simulink model "gm_HDL_pfc_gold_fi_og_vnl"  (R2024b)
settings: Solver=FixedStepDiscrete  StartTime=0.0  StopTime=.2  RelTol=1e-3
InitFcn:
  | fidelity_pfc_vals;
  | nbits=(2^12)-2;
  | load('C:\Users\Angel\Desktop\hil\pfc3ph\matlab\sim\sschdl\pfc_desktop\stateSpaceParameters.mat');
undefined symbols (not defined in the file or in its folder): a, b, c, DiscIntNeverNeededParam, fsw, Gs, s, stateSpaceParameters_1, t_ss, tsw
libraries: simulink x47, hdlmdlgenlib x24, hdlsllib x10, mcbcontrolslib x5, dspsrcs4 x3, slpidlib x2, hdlssclib x2, spsSVPWMGenerator2LevelLib x1, spsPLL3phLib x1, fillib x1
(part 1 of 5)
settings Model: Creator=angro  LastModifiedBy=Angel
settings OptimizationCC: BlockReduction=off  ConditionallyExecuteInputs=off  DefaultParameterBehavior=Inlined  InheritOutputTypeSmallerThanSingle=on  DefaultUnderspecifiedDataType=single
settings DebuggingCC: SignalRangeChecking=warning  AlgebraicLoopMsg=none  ArtificialAlgebraicLoopMsg=error  InheritedTsInSrcMsg=none  SingleTaskRateTransMsg=error  UnconnectedInputMsg=warning  UnconnectedOutputMsg=warning  UnconnectedLineMsg=warning
settings HardwareCC: ProdBitPerPointer=32  ProdBitPerSizeT=32  ProdBitPerPtrDiffT=32  ProdLargestAtomicFloat=None  ProdIntDivRoundTo=Undefined  ProdEndianess=Unspecified  ProdWordSize=32  ProdHWDeviceType=ASIC/FPGA->ASIC/FPGA  TargetBitPerPointer=64  TargetBitPerSizeT=64  TargetBitPerPtrDiffT=64  TargetLongLongMode=on  TargetIntDivRoundTo=Zero  TargetEndianess=LittleEndian  TargetWordSize=64  TargetHWDeviceType=Custom Processor->MATLAB Host Computer  ProdEqTarget=off

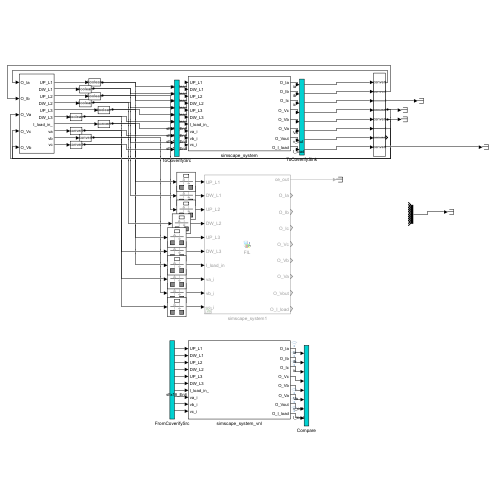
[thumbnail: Simulink's stored preview of the top-level diagram]
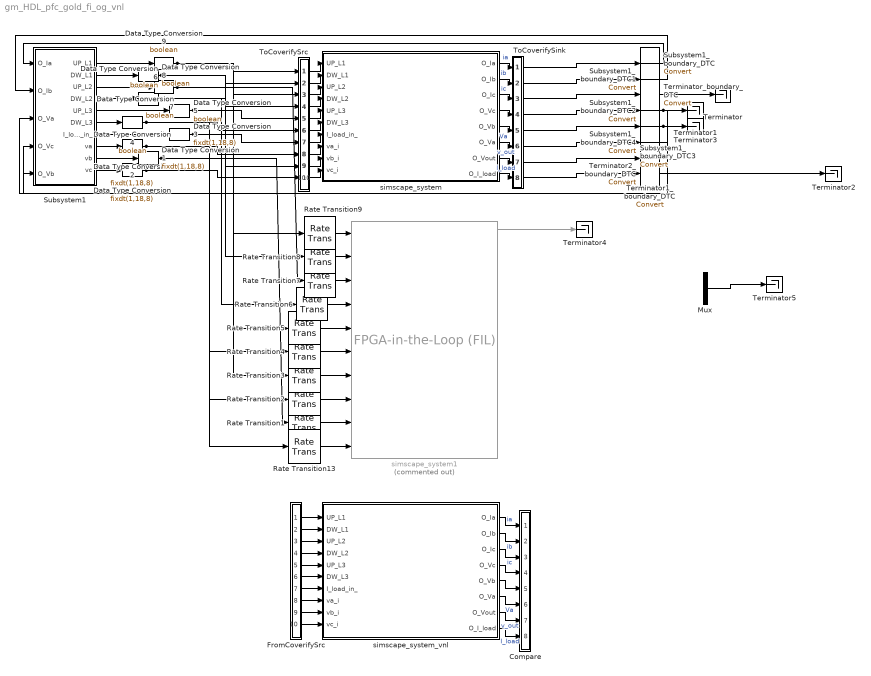
== system gm_HDL_pfc_gold_fi_og_vnl ==
  Compare : Subsystem
      mask Display: disp('')
  Data Type Conversion{,1..3} (4 alike) : DataTypeConversion  OutDataTypeStr=fixdt(1,18,8)  SaturateOnIntegerOverflow=off  RndMeth=Floor
  Data Type Conversion{4..9} (6 alike) : DataTypeConversion  OutDataTypeStr=boolean  SaturateOnIntegerOverflow=off  RndMeth=Floor
  FromCoverifySrc : Subsystem
      mask Display: disp('')
  Mux : Mux  Inputs=9
  Rate Transition{1..9,13} (10 alike) : RateTransition
  Subsystem1 : Subsystem
  Subsystem1_boundary_DTC{,1..4} (5 alike) : DataTypeConversion
  Terminator{,1..5} (6 alike) : Terminator
  Terminator1_boundary_DTC : DataTypeConversion
  Terminator2_boundary_DTC : DataTypeConversion
  Terminator_boundary_DTC : DataTypeConversion
  ToCoverifySink : Subsystem
      mask Display: disp('')
  ToCoverifySrc : Subsystem
      mask Display: disp('')
  simscape_system : Subsystem
  simscape_system1 : fillib/FPGA-in-the-Loop (FIL)  Commented=on  ForceInterfaceUpdate=0.086758
  simscape_system_vnl : Subsystem
  wires:
  Subsystem1/7(I_load_in_) -> Data Type Conversion3/1
  Subsystem1/1(UP_L1) -> Data Type Conversion9/1
  Subsystem1/2(DW_L1) -> Data Type Conversion8/1
  Subsystem1/3(UP_L2) -> Data Type Conversion7/1
  Subsystem1/4(DW_L2) -> Data Type Conversion6/1
  Subsystem1/5(UP_L3) -> Data Type Conversion5/1
  Subsystem1/6(DW_L3) -> Data Type Conversion4/1
  Subsystem1/8(va) -> Data Type Conversion2/1
  Subsystem1/9(vb) -> Data Type Conversion1/1
  Subsystem1/10(vc) -> Data Type Conversion/1
  Data Type Conversion/1 -> Rate Transition13/1, ToCoverifySrc/10(in10)
  Data Type Conversion1/1 -> Rate Transition1/1, ToCoverifySrc/9(in9)
  Data Type Conversion2/1 -> Rate Transition2/1, ToCoverifySrc/8(in8)
  Data Type Conversion3/1 -> Rate Transition3/1, ToCoverifySrc/7(in7)
  Data Type Conversion4/1 -> Rate Transition4/1, ToCoverifySrc/6(in6)
  Data Type Conversion5/1 -> Rate Transition5/1, ToCoverifySrc/5(in5)
  Data Type Conversion6/1 -> Rate Transition6/1, ToCoverifySrc/4(in4)
  Data Type Conversion7/1 -> Rate Transition7/1, ToCoverifySrc/3(in3)
  Data Type Conversion8/1 -> Rate Transition8/1, ToCoverifySrc/2(in2)
  Data Type Conversion9/1 -> Rate Transition9/1, ToCoverifySrc/1(in1)
  Terminator_boundary_DTC/1 -> Terminator/1
  Terminator2_boundary_DTC/1 -> Terminator2/1
  Subsystem1_boundary_DTC/1 -> Subsystem1/1(O_Ia)
  Subsystem1_boundary_DTC1/1 -> Subsystem1/2(O_Ib)
  Subsystem1_boundary_DTC2/1 -> Terminator1/1, Subsystem1/4(O_Vc)
  Subsystem1_boundary_DTC3/1 -> Terminator3/1, Subsystem1/5(O_Vb)
  Subsystem1_boundary_DTC4/1 -> Subsystem1/3(O_Va)
  simscape_system1/1 -> Terminator4/1
  Rate Transition13/1 -> simscape_system1/10
  Rate Transition1/1 -> simscape_system1/9
  Rate Transition2/1 -> simscape_system1/8
  Rate Transition3/1 -> simscape_system1/7
  Rate Transition4/1 -> simscape_system1/6
  Rate Transition5/1 -> simscape_system1/5
  Rate Transition6/1 -> simscape_system1/4
  Rate Transition7/1 -> simscape_system1/3
  Rate Transition8/1 -> simscape_system1/2
  Rate Transition9/1 -> simscape_system1/1
  Mux/1 -> Terminator5/1
  ToCoverifySrc/1(out1) -> simscape_system/1(UP_L1)
  ToCoverifySrc/2(out2) -> simscape_system/2(DW_L1)
  ToCoverifySrc/3(out3) -> simscape_system/3(UP_L2)
  ToCoverifySrc/4(out4) -> simscape_system/4(DW_L2)
  ToCoverifySrc/5(out5) -> simscape_system/5(UP_L3)
  ToCoverifySrc/6(out6) -> simscape_system/6(DW_L3)
  ToCoverifySrc/7(out7) -> simscape_system/7(I_load_in_)
  ToCoverifySrc/8(out8) -> simscape_system/8(va_i)
  ToCoverifySrc/9(out9) -> simscape_system/9(vb_i)
  ToCoverifySrc/10(out10) -> simscape_system/10(vc_i)
  simscape_system/1(O_Ia) -> ToCoverifySink/1(in1)  "ia"
  simscape_system/2(O_Ib) -> ToCoverifySink/2(in2)  "ib"
  simscape_system/3(O_Ic) -> ToCoverifySink/3(in3)  "ic"
  simscape_system/4(O_Vc) -> ToCoverifySink/4(in4)
  simscape_system/5(O_Vb) -> ToCoverifySink/5(in5)
  simscape_system/6(O_Va) -> ToCoverifySink/6(in6)  "Va"
  simscape_system/7(O_Vout) -> ToCoverifySink/7(in7)  "v_out"
  simscape_system/8(O_I_load) -> ToCoverifySink/8(in8)  "I_load"
  ToCoverifySink/1(out1) -> Subsystem1_boundary_DTC/1
  ToCoverifySink/2(out2) -> Subsystem1_boundary_DTC1/1
  ToCoverifySink/3(out3) -> Terminator_boundary_DTC/1
  ToCoverifySink/4(out4) -> Subsystem1_boundary_DTC2/1
  ToCoverifySink/5(out5) -> Subsystem1_boundary_DTC3/1
  ToCoverifySink/6(out6) -> Subsystem1_boundary_DTC4/1
  ToCoverifySink/7(out7) -> Terminator1_boundary_DTC/1
  ToCoverifySink/8(out8) -> Terminator2_boundary_DTC/1
  FromCoverifySrc/1(out1) -> simscape_system_vnl/1(UP_L1)
  FromCoverifySrc/2(out2) -> simscape_system_vnl/2(DW_L1)
  FromCoverifySrc/3(out3) -> simscape_system_vnl/3(UP_L2)
  FromCoverifySrc/4(out4) -> simscape_system_vnl/4(DW_L2)
  FromCoverifySrc/5(out5) -> simscape_system_vnl/5(UP_L3)
  FromCoverifySrc/6(out6) -> simscape_system_vnl/6(DW_L3)
  FromCoverifySrc/7(out7) -> simscape_system_vnl/7(I_load_in_)
  FromCoverifySrc/8(out8) -> simscape_system_vnl/8(va_i)
  FromCoverifySrc/9(out9) -> simscape_system_vnl/9(vb_i)
  FromCoverifySrc/10(out10) -> simscape_system_vnl/10(vc_i)
  simscape_system_vnl/1(O_Ia) -> Compare/1(in1)  "ia"
  simscape_system_vnl/2(O_Ib) -> Compare/2(in2)  "ib"
  simscape_system_vnl/3(O_Ic) -> Compare/3(in3)  "ic"
  simscape_system_vnl/4(O_Vc) -> Compare/4(in4)
  simscape_system_vnl/5(O_Vb) -> Compare/5(in5)
  simscape_system_vnl/6(O_Va) -> Compare/6(in6)  "Va"
  simscape_system_vnl/7(O_Vout) -> Compare/7(in7)  "v_out"
  simscape_system_vnl/8(O_I_load) -> Compare/8(in8)  "I_load"

== system gm_HDL_pfc_gold_fi_og_vnl/Compare ==
  in1 : Inport
  in2 : Inport  Port=2
  in3 : Inport  Port=3
  in4 : Inport  Port=4
  in5 : Inport  Port=5
  in6 : Inport  Port=6
  in7 : Inport  Port=7
  in8 : Inport  Port=8
  Assert_O_I_load : Subsystem
  Assert_O_Ia : Subsystem
  Assert_O_Ib : Subsystem
  Assert_O_Ic : Subsystem
  Assert_O_Va : Subsystem
  Assert_O_Vb : Subsystem
  Assert_O_Vc : Subsystem
  Assert_O_Vout : Subsystem
  CleanupScopes : Subsystem
      settings: OpenFcn=|
      | blkName = gcb; %self block
      | idx = regexp(blkName, '/CleanupScopes$', 'once');
      | blkParent = blkName(1:idx-1);
      | blks=find_system(blkParent, 'LookUnderMasks', 'all','blocktype', 'Scope');
      | for itr = 1:length(blks)
      | 	 hScopeCfg = get_param(blks{itr},'ScopeConfiguration');
      | 	 hScopeCfg.Visible = ~ hScopeCfg.Visible;
      | end
      | drawnow;
      mask Display: fprintf(message('hdlcoder:cosim:vnl_dblclick').getString());
  Enable : Subsystem
      settings: OpenFcn=|
      | blkName = gcb;
      | idx = regexp(blkName, '/Enable$', 'once');
      | blkParent = blkName(1:idx-1);
      | blks=find_system(blkParent, 'LookUnderMasks', 'all','blocktype', 'Assertion');
      | e = get_param(blks{1}, 'Enabled');
      | if strcmp(e, 'on'), f= 'off';, else, f = 'on';, end
      | for ii=1:length(blks), set_param(blks{ii}, 'Enabled', f);, end
      | set_param(gcb, 'MaskDisplay',['fprintf(message(''hdlcoder:cosim:vnl_dblclick_assertions'',','''',upper(e),'''',').getString())']);
      mask Display: fprintf(message('hdlcoder:cosim:vnl_dblclick_assertions','OFF').getString());
  wires:
  in1/1 -> Assert_O_Ia/1(cosim)
  [out1] -> Assert_O_Ia/2(dut)
  in2/1 -> Assert_O_Ib/1(cosim)
  [out2] -> Assert_O_Ib/2(dut)
  in3/1 -> Assert_O_Ic/1(cosim)
  [out3] -> Assert_O_Ic/2(dut)
  in4/1 -> Assert_O_Vc/1(cosim)
  [out4] -> Assert_O_Vc/2(dut)
  in5/1 -> Assert_O_Vb/1(cosim)
  [out5] -> Assert_O_Vb/2(dut)
  in6/1 -> Assert_O_Va/1(cosim)
  [out6] -> Assert_O_Va/2(dut)
  in7/1 -> Assert_O_Vout/1(cosim)
  [out7] -> Assert_O_Vout/2(dut)
  in8/1 -> Assert_O_I_load/1(cosim)
  [out8] -> Assert_O_I_load/2(dut)

== system gm_HDL_pfc_gold_fi_og_vnl/FromCoverifySrc ==
  out1 : Outport
  out2 : Outport  Port=2
  out3 : Outport  Port=3
  out4 : Outport  Port=4
  out5 : Outport  Port=5
  out6 : Outport  Port=6
  out7 : Outport  Port=7
  out8 : Outport  Port=8
  out9 : Outport  Port=9
  out10 : Outport  Port=10
  wires:
  [in1] -> out1/1
  [in2] -> out2/1
  [in3] -> out3/1
  [in4] -> out4/1
  [in5] -> out5/1
  [in6] -> out6/1
  [in7] -> out7/1
  [in8] -> out8/1
  [in9] -> out9/1
  [in10] -> out10/1

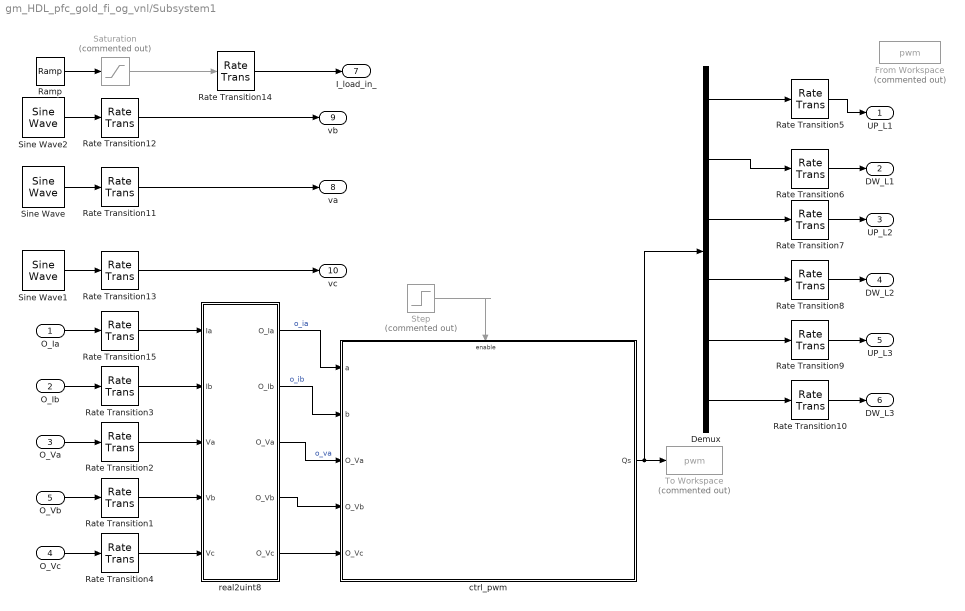
== system gm_HDL_pfc_gold_fi_og_vnl/Subsystem1 ==
  O_Ia : Inport
  O_Ib : Inport  Port=2
  O_Va : Inport  Port=3
  O_Vc : Inport  Port=4
  O_Vb : Inport  Port=5
  Demux : Demux  Outputs=6
  From Workspace : FromWorkspace  Commented=on  VariableName=pwm  SampleTime=t_ss  Interpolate=off  ZeroCross=off  OutputAfterFinalValue=Holding final value
  Ramp : simulink/Sources/Ramp  slope=1/50  start=2/50  InitialOutput=0
  Rate Transition{1..13,15} (14 alike) : RateTransition
  Rate Transition14 : RateTransition  OutPortSampleTime=t_ss
  Saturation : Saturate  Commented=on  UpperLimit=2
  Sine Wave : dspsrcs4/Sine Wave  Amplitude=325  Frequency=50  Phase=0  SampleMode=Discrete  OutComplex=Real  CompMethod=Table lookup  TableSize=Speed  SampleTime=tsw  SamplesPerFrame=1  ResetState=Restart at time zero  OutputFrames=off  dataType=double  wordLen=16  udDataType=sfix(16)  fracBitsMode=Best precision  numFracBits=15  OutDataTypeStr=double  LastOutDataTypeStr=double
  Sine Wave1 : dspsrcs4/Sine Wave  Amplitude=325  Frequency=50  Phase=2*pi/3  SampleMode=Discrete  OutComplex=Real  CompMethod=Table lookup  TableSize=Speed  SampleTime=tsw  SamplesPerFrame=1  ResetState=Restart at time zero  OutputFrames=off  dataType=double  wordLen=16  udDataType=sfix(16)  fracBitsMode=Best precision  numFracBits=15  OutDataTypeStr=double  LastOutDataTypeStr=double
  Sine Wave2 : dspsrcs4/Sine Wave  Amplitude=325  Frequency=50  Phase=-2*pi/3  SampleMode=Discrete  OutComplex=Real  CompMethod=Table lookup  TableSize=Speed  SampleTime=tsw  SamplesPerFrame=1  ResetState=Restart at time zero  OutputFrames=off  dataType=double  wordLen=16  udDataType=sfix(16)  fracBitsMode=Best precision  numFracBits=15  OutDataTypeStr=double  LastOutDataTypeStr=double
  Step : Step  Commented=on  Time=2/50  SampleTime=0
  To Workspace : ToWorkspace  Commented=on  VariableName=pwm  SaveFormat=Timeseries  SampleTime=-1
  ctrl_pwm : Subsystem
  real2uint8 : Subsystem
  UP_L1 : Outport
  DW_L1 : Outport  Port=2
  UP_L2 : Outport  Port=3
  DW_L2 : Outport  Port=4
  UP_L3 : Outport  Port=5
  DW_L3 : Outport  Port=6
  I_load_in_ : Outport  Port=7
  va : Outport  Port=8
  vb : Outport  Port=9
  vc : Outport  Port=10
  wires:
  Ramp/1 -> Saturation/1
  Rate Transition15/1 -> real2uint8/1(Ia)
  Sine Wave2/1 -> Rate Transition12/1
  Saturation/1 -> Rate Transition14/1
  Sine Wave1/1 -> Rate Transition13/1
  Rate Transition8/1 -> DW_L2/1
  Sine Wave/1 -> Rate Transition11/1
  O_Ib/1 -> Rate Transition3/1
  O_Vb/1 -> Rate Transition1/1
  O_Va/1 -> Rate Transition2/1
  O_Ia/1 -> Rate Transition15/1
  O_Vc/1 -> Rate Transition4/1
  Rate Transition2/1 -> real2uint8/3(Va)
  Rate Transition12/1 -> vb/1
  Rate Transition3/1 -> real2uint8/2(Ib)
  Rate Transition11/1 -> va/1
  Rate Transition1/1 -> real2uint8/4(Vb)
  Rate Transition13/1 -> vc/1
  Rate Transition4/1 -> real2uint8/5(Vc)
  Rate Transition10/1 -> DW_L3/1
  Rate Transition14/1 -> I_load_in_/1
  Step/1 -> ctrl_pwm/Enable
  real2uint8/4(O_Vb) -> ctrl_pwm/4(O_Vb)
  real2uint8/1(O_Ia) -> ctrl_pwm/1(a)  "o_ia"
  real2uint8/2(O_Ib) -> ctrl_pwm/2(b)  "o_ib"
  real2uint8/3(O_Va) -> ctrl_pwm/3(O_Va)  "o_va"
  real2uint8/5(O_Vc) -> ctrl_pwm/5(O_Vc)
  ctrl_pwm/1(Qs) -> Demux/1, To Workspace/1
  Demux/5 -> Rate Transition9/1
  Demux/1 -> Rate Transition5/1
  Demux/6 -> Rate Transition10/1
  Demux/2 -> Rate Transition6/1
  Demux/3 -> Rate Transition7/1
  Demux/4 -> Rate Transition8/1
  Rate Transition5/1 -> UP_L1/1
  Rate Transition6/1 -> DW_L1/1
  Rate Transition7/1 -> UP_L2/1
  Rate Transition9/1 -> UP_L3/1

== system gm_HDL_pfc_gold_fi_og_vnl/ToCoverifySink ==
  in1 : Inport
  in2 : Inport  Port=2
  in3 : Inport  Port=3
  in4 : Inport  Port=4
  in5 : Inport  Port=5
  in6 : Inport  Port=6
  in7 : Inport  Port=7
  in8 : Inport  Port=8
  out1 : Outport
  out2 : Outport  Port=2
  out3 : Outport  Port=3
  out4 : Outport  Port=4
  out5 : Outport  Port=5
  out6 : Outport  Port=6
  out7 : Outport  Port=7
  out8 : Outport  Port=8
  tag scope: out1=global, out2=global, out3=global, out4=global, out5=global, out6=global, out7=global, out8=global
  wires:
  in1/1 -> out1/1, [out1]
  in2/1 -> out2/1, [out2]
  in3/1 -> out3/1, [out3]
  in4/1 -> out4/1, [out4]
  in5/1 -> out5/1, [out5]
  in6/1 -> out6/1, [out6]
  in7/1 -> out7/1, [out7]
  in8/1 -> out8/1, [out8]

== system gm_HDL_pfc_gold_fi_og_vnl/ToCoverifySrc ==
  in1 : Inport
  in2 : Inport  Port=2
  in3 : Inport  Port=3
  in4 : Inport  Port=4
  in5 : Inport  Port=5
  in6 : Inport  Port=6
  in7 : Inport  Port=7
  in8 : Inport  Port=8
  in9 : Inport  Port=9
  in10 : Inport  Port=10
  out1 : Outport
  out2 : Outport  Port=2
  out3 : Outport  Port=3
  out4 : Outport  Port=4
  out5 : Outport  Port=5
  out6 : Outport  Port=6
  out7 : Outport  Port=7
  out8 : Outport  Port=8
  out9 : Outport  Port=9
  out10 : Outport  Port=10
  tag scope: in10=global, in1=global, in2=global, in3=global, in4=global, in5=global, in6=global, in7=global, in8=global, in9=global
  wires:
  in1/1 -> out1/1, [in1]
  in2/1 -> out2/1, [in2]
  in3/1 -> out3/1, [in3]
  in4/1 -> out4/1, [in4]
  in5/1 -> out5/1, [in5]
  in6/1 -> out6/1, [in6]
  in7/1 -> out7/1, [in7]
  in8/1 -> out8/1, [in8]
  in9/1 -> out9/1, [in9]
  in10/1 -> out10/1, [in10]

== system gm_HDL_pfc_gold_fi_og_vnl/simscape_system ==
  UP_L1 : Inport  OutDataTypeStr=boolean  PortDimensions=1  SampleTime=5.12820512820513e-07
  DW_L1 : Inport  Port=2  OutDataTypeStr=boolean  PortDimensions=1  SampleTime=5.12820512820513e-07
  UP_L2 : Inport  Port=3  OutDataTypeStr=boolean  PortDimensions=1  SampleTime=5.12820512820513e-07
  DW_L2 : Inport  Port=4  OutDataTypeStr=boolean  PortDimensions=1  SampleTime=5.12820512820513e-07
  UP_L3 : Inport  Port=5  OutDataTypeStr=boolean  PortDimensions=1  SampleTime=5.12820512820513e-07
  DW_L3 : Inport  Port=6  OutDataTypeStr=boolean  PortDimensions=1  SampleTime=5.12820512820513e-07
  I_load_in_ : Inport  Port=7  OutDataTypeStr=fixdt(1, 18, 8)  PortDimensions=1  SampleTime=5.12820512820513e-07
  va_i : Inport  Port=8  OutDataTypeStr=fixdt(1, 18, 8)  PortDimensions=1  SampleTime=5.12820512820513e-07  LockScale=on
  vb_i : Inport  Port=9  OutDataTypeStr=fixdt(1, 18, 8)  PortDimensions=1  SampleTime=5.12820512820513e-07  LockScale=on
  vc_i : Inport  Port=10  OutDataTypeStr=fixdt(1, 18, 8)  PortDimensions=1  SampleTime=5.12820512820513e-07  LockScale=on
  simscape_system : Subsystem
  t{,1..7} (8 alike) : RateTransition  InitialCondition=double(0)  OutPortSampleTimeOpt=Multiple of input port sample time  OutPortSampleTimeMultiple=37
  O_Ia : Outport  SampleTime=5.12820512820513e-07
  O_Ib : Outport  Port=2  SampleTime=5.12820512820513e-07
  O_Ic : Outport  Port=3  SampleTime=5.12820512820513e-07
  O_Vc : Outport  Port=4  SampleTime=5.12820512820513e-07
  O_Vb : Outport  Port=5  SampleTime=5.12820512820513e-07
  O_Va : Outport  Port=6  SampleTime=5.12820512820513e-07
  O_Vout : Outport  Port=7  SampleTime=5.12820512820513e-07
  O_I_load : Outport  Port=8  SampleTime=5.12820512820513e-07
  wires:
  t6/1 -> O_I_load/1
  t5/1 -> O_Vout/1
  t4/1 -> O_Va/1
  t3/1 -> O_Vb/1
  t2/1 -> O_Vc/1
  t1/1 -> O_Ic/1
  t/1 -> O_Ib/1
  t7/1 -> O_Ia/1
  simscape_system/8(O_I_load) -> t6/1
  simscape_system/7(O_Vout) -> t5/1
  simscape_system/6(O_Va) -> t4/1
  simscape_system/5(O_Vb) -> t3/1
  simscape_system/4(O_Vc) -> t2/1
  simscape_system/3(O_Ic) -> t1/1
  simscape_system/2(O_Ib) -> t/1
  simscape_system/1(O_Ia) -> t7/1
  vc_i/1 -> simscape_system/10(vc_i)
  vb_i/1 -> simscape_system/9(vb_i)
  I_load_in_/1 -> simscape_system/7(I_load_in_)
  va_i/1 -> simscape_system/8(va_i)
  UP_L1/1 -> simscape_system/1(UP_L1)
  DW_L1/1 -> simscape_system/2(DW_L1)
  UP_L2/1 -> simscape_system/3(UP_L2)
  DW_L2/1 -> simscape_system/4(DW_L2)
  UP_L3/1 -> simscape_system/5(UP_L3)
  DW_L3/1 -> simscape_system/6(DW_L3)

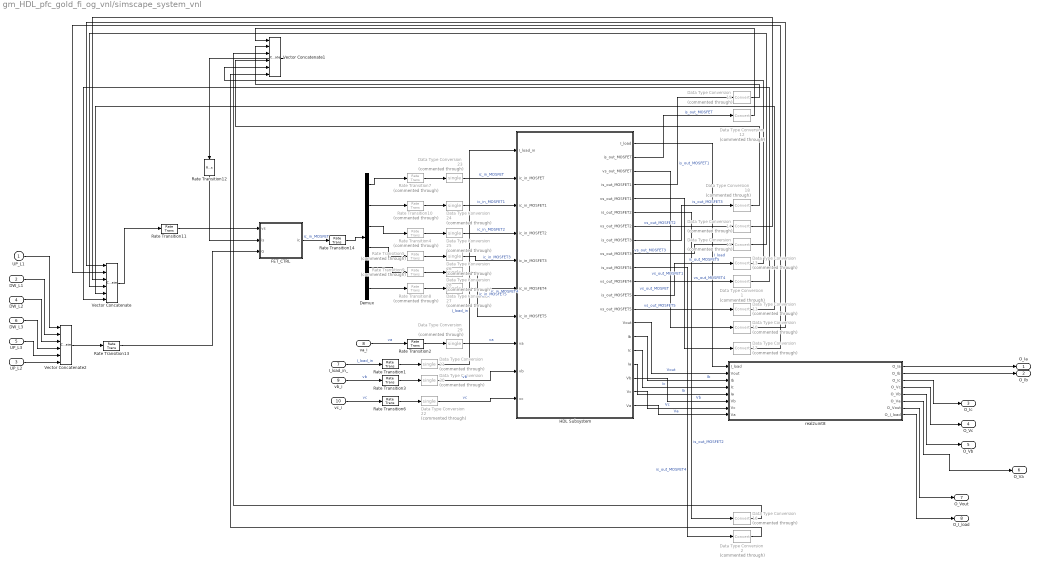
== system gm_HDL_pfc_gold_fi_og_vnl/simscape_system_vnl ==
  UP_L1 : Inport
  DW_L1 : Inport  Port=2
  UP_L2 : Inport  Port=3
  DW_L2 : Inport  Port=4
  UP_L3 : Inport  Port=5
  DW_L3 : Inport  Port=6
  I_load_in_ : Inport  Port=7  OutDataTypeStr=fixdt(1,18,8)
  va_i : Inport  Port=8  LockScale=on
  vb_i : Inport  Port=9  LockScale=on
  vc_i : Inport  Port=10  LockScale=on
  Data Type Conversion{1..2,10..19} (12 alike) : DataTypeConversion  Commented=through  RndMeth=Nearest  SaturateOnIntegerOverflow=off  LockScale=on
  Data Type Conversion{21..30} (10 alike) : DataTypeConversion  Commented=through  OutDataTypeStr=single  RndMeth=Nearest  SaturateOnIntegerOverflow=off
  Demux : Demux  Outputs=6
  FET_CTRL : Subsystem
  HDL Subsystem : Subsystem
  Rate Transition{1..3,6,11..13} (7 alike) : RateTransition  OutPortSampleTime=t_ss
  Rate Transition{4..5,7..10} (6 alike) : RateTransition  Commented=through  OutPortSampleTime=t_ss
  Rate Transition14 : RateTransition  Integrity=off  OutPortSampleTime=t_ss
  Vector Concatenate : Concatenate  NumInputs=6
  Vector Concatenate1 : Concatenate  NumInputs=6
  Vector Concatenate2 : Concatenate  NumInputs=6
  real2uint8 : Subsystem
  O_Ia : Outport
  O_Ib : Outport  Port=2
  O_Ic : Outport  Port=3
  O_Vc : Outport  Port=4
  O_Vb : Outport  Port=5
  O_Va : Outport  Port=6
  O_Vout : Outport  Port=7
  O_I_load : Outport  Port=8
  wires:
  real2uint8/6(O_Va) -> O_Va/1
  real2uint8/2(O_Ib) -> O_Ib/1
  real2uint8/1(O_Ia) -> O_Ia/1
  Rate Transition12/1 -> FET_CTRL/2(is)
  Rate Transition11/1 -> FET_CTRL/1(vs)
  Rate Transition14/1 -> Demux/1
  Vector Concatenate1/1 -> Rate Transition12/1
  Vector Concatenate/1 -> Rate Transition11/1
  Rate Transition13/1 -> FET_CTRL/3(G)
  real2uint8/7(O_Vout) -> O_Vout/1
  Data Type Conversion2/1 -> Vector Concatenate1/6
  Data Type Conversion16/1 -> Vector Concatenate1/3
  real2uint8/8(O_I_load) -> O_I_load/1
  real2uint8/5(O_Vb) -> O_Vb/1
  real2uint8/4(O_Vc) -> O_Vc/1
  real2uint8/3(O_Ic) -> O_Ic/1
  Data Type Conversion17/1 -> Vector Concatenate/2
  Data Type Conversion10/1 -> Vector Concatenate/1
  Data Type Conversion11/1 -> Vector Concatenate/5
  Data Type Conversion1/1 -> Vector Concatenate/6
  Data Type Conversion13/1 -> Vector Concatenate1/5
  Data Type Conversion15/1 -> Vector Concatenate/4
  Data Type Conversion14/1 -> Vector Concatenate/3
  Data Type Conversion12/1 -> Vector Concatenate1/1
  HDL Subsystem/11(vs_out_MOSFET4) -> Data Type Conversion1/1  "vs_out_MOSFET4"
  HDL Subsystem/12(is_out_MOSFET5) -> Data Type Conversion13/1  "is_out_MOSFET5"
  HDL Subsystem/9(vs_out_MOSFET3) -> Data Type Conversion15/1  "vs_out_MOSFET3"
  HDL Subsystem/10(is_out_MOSFET4) -> Data Type Conversion2/1  "is_out_MOSFET4"
  HDL Subsystem/7(vs_out_MOSFET2) -> Data Type Conversion14/1  "vs_out_MOSFET2"
  HDL Subsystem/8(is_out_MOSFET3) -> Data Type Conversion18/1  "is_out_MOSFET3"
  HDL Subsystem/5(vs_out_MOSFET1) -> Data Type Conversion17/1  "vs_out_MOSFET1"
  HDL Subsystem/6(is_out_MOSFET2) -> Data Type Conversion16/1  "is_out_MOSFET2"
  Data Type Conversion22/1 -> HDL Subsystem/10(vc)  "vc"
  Data Type Conversion30/1 -> HDL Subsystem/9(vb)  "vb"
  HDL Subsystem/3(vs_out_MOSFET) -> Data Type Conversion10/1  "vs_out_MOSFET"
  HDL Subsystem/4(is_out_MOSFET1) -> Data Type Conversion19/1  "is_out_MOSFET1"
  Data Type Conversion29/1 -> HDL Subsystem/8(va)  "va"
  Data Type Conversion27/1 -> HDL Subsystem/6(ic_in_MOSFET4)  "ic_in_MOSFET4"
  Data Type Conversion28/1 -> HDL Subsystem/7(ic_in_MOSFET5)  "ic_in_MOSFET5"
  Data Type Conversion26/1 -> HDL Subsystem/5(ic_in_MOSFET3)  "ic_in_MOSFET3"
  Data Type Conversion25/1 -> HDL Subsystem/4(ic_in_MOSFET2)  "ic_in_MOSFET2"
  Data Type Conversion23/1 -> HDL Subsystem/2(ic_in_MOSFET)  "ic_in_MOSFET"
  Rate Transition6/1 -> Data Type Conversion22/1
  Data Type Conversion19/1 -> Vector Concatenate1/2
  Rate Transition3/1 -> Data Type Conversion30/1
  Rate Transition1/1 -> Data Type Conversion21/1
  Data Type Conversion24/1 -> HDL Subsystem/3(ic_in_MOSFET1)  "ic_in_MOSFET1"
  Rate Transition2/1 -> Data Type Conversion29/1
  Data Type Conversion18/1 -> Vector Concatenate1/4
  Rate Transition8/1 -> Data Type Conversion27/1
  Rate Transition9/1 -> Data Type Conversion28/1
  Data Type Conversion21/1 -> HDL Subsystem/1(I_load_in)  "I_load_in"
  Rate Transition5/1 -> Data Type Conversion26/1
  Rate Transition4/1 -> Data Type Conversion25/1
  Rate Transition10/1 -> Data Type Conversion24/1
  vc_i/1 -> Rate Transition6/1  "vc"
  Demux/5 -> Rate Transition9/1
  Demux/6 -> Rate Transition8/1
  vb_i/1 -> Rate Transition3/1  "vb"
  Demux/3 -> Rate Transition4/1
  Demux/4 -> Rate Transition5/1
  va_i/1 -> Rate Transition2/1  "va"
  Rate Transition7/1 -> Data Type Conversion23/1
  Demux/1 -> Rate Transition7/1
  Demux/2 -> Rate Transition10/1
  I_load_in_/1 -> Rate Transition1/1  "I_load_in"
  FET_CTRL/1(ic) -> Rate Transition14/1  "ic_in_MOSFET"
  Vector Concatenate2/1 -> Rate Transition13/1
  HDL Subsystem/1(I_load) -> real2uint8/1(I_load)  "I_load"
  HDL Subsystem/2(is_out_MOSFET) -> Data Type Conversion12/1  "is_out_MOSFET"
  UP_L2/1 -> Vector Concatenate2/6
  HDL Subsystem/17(Ia) -> real2uint8/5(Ia)  "Ia"
  HDL Subsystem/18(Vb) -> real2uint8/6(Vb)  "Vb"
  UP_L3/1 -> Vector Concatenate2/5
  DW_L3/1 -> Vector Concatenate2/4
  DW_L2/1 -> Vector Concatenate2/3
  HDL Subsystem/19(Vc) -> real2uint8/7(Vc)  "Vc"
  HDL Subsystem/20(Va) -> real2uint8/8(Va)  "Va"
  DW_L1/1 -> Vector Concatenate2/2
  HDL Subsystem/15(Ib) -> real2uint8/3(Ib)  "Ib"
  HDL Subsystem/16(Ic) -> real2uint8/4(Ic)  "Ic"
  UP_L1/1 -> Vector Concatenate2/1
  HDL Subsystem/13(vs_out_MOSFET5) -> Data Type Conversion11/1  "vs_out_MOSFET5"
  HDL Subsystem/14(Vout) -> real2uint8/2(Vout)  "Vout"

== system gm_HDL_pfc_gold_fi_og_vnl/Compare/Assert_O_I_load ==
  cosim : Inport
  dut : Inport  Port=2
  AssertEq : Assertion  StopWhenAssertionFail=off
  Compare To Zero : simulink/Logic and Bit Operations/Compare To Zero  relop===  OutDataTypeStr=boolean
  Relational Operator : RelationalOperator  Operator===  OutDataTypeStr=boolean  InputSameDT=off
  compare: O_I_load : Scope  NumInputPorts=3
  wires:
  Compare To Zero/1 -> compare: O_I_load/3  "err"
  Relational Operator/1 -> Compare To Zero/1, AssertEq/1
  cosim/1 -> compare: O_I_load/1, Relational Operator/1  "cosim"
  dut/1 -> compare: O_I_load/2, Relational Operator/2  "dut ref"

== system gm_HDL_pfc_gold_fi_og_vnl/Compare/Assert_O_Ia ==
  cosim : Inport
  dut : Inport  Port=2
  AssertEq : Assertion  StopWhenAssertionFail=off
  Compare To Zero : simulink/Logic and Bit Operations/Compare To Zero  relop===  OutDataTypeStr=boolean
  Relational Operator : RelationalOperator  Operator===  OutDataTypeStr=boolean  InputSameDT=off
  compare: O_Ia : Scope  NumInputPorts=3
  wires:
  Compare To Zero/1 -> compare: O_Ia/3  "err"
  Relational Operator/1 -> Compare To Zero/1, AssertEq/1
  cosim/1 -> compare: O_Ia/1, Relational Operator/1  "cosim"
  dut/1 -> compare: O_Ia/2, Relational Operator/2  "dut ref"

== system gm_HDL_pfc_gold_fi_og_vnl/Compare/Assert_O_Ib ==
  cosim : Inport
  dut : Inport  Port=2
  AssertEq : Assertion  StopWhenAssertionFail=off
  Compare To Zero : simulink/Logic and Bit Operations/Compare To Zero  relop===  OutDataTypeStr=boolean
  Relational Operator : RelationalOperator  Operator===  OutDataTypeStr=boolean  InputSameDT=off
  compare: O_Ib : Scope  NumInputPorts=3
  wires:
  Compare To Zero/1 -> compare: O_Ib/3  "err"
  Relational Operator/1 -> Compare To Zero/1, AssertEq/1
  cosim/1 -> compare: O_Ib/1, Relational Operator/1  "cosim"
  dut/1 -> compare: O_Ib/2, Relational Operator/2  "dut ref"

== system gm_HDL_pfc_gold_fi_og_vnl/Compare/Assert_O_Ic ==
  cosim : Inport
  dut : Inport  Port=2
  AssertEq : Assertion  StopWhenAssertionFail=off
  Compare To Zero : simulink/Logic and Bit Operations/Compare To Zero  relop===  OutDataTypeStr=boolean
  Relational Operator : RelationalOperator  Operator===  OutDataTypeStr=boolean  InputSameDT=off
  compare: O_Ic : Scope  NumInputPorts=3
  wires:
  Compare To Zero/1 -> compare: O_Ic/3  "err"
  Relational Operator/1 -> Compare To Zero/1, AssertEq/1
  cosim/1 -> compare: O_Ic/1, Relational Operator/1  "cosim"
  dut/1 -> compare: O_Ic/2, Relational Operator/2  "dut ref"

== system gm_HDL_pfc_gold_fi_og_vnl/Compare/Assert_O_Va ==
  cosim : Inport
  dut : Inport  Port=2
  AssertEq : Assertion  StopWhenAssertionFail=off
  Compare To Zero : simulink/Logic and Bit Operations/Compare To Zero  relop===  OutDataTypeStr=boolean
  Relational Operator : RelationalOperator  Operator===  OutDataTypeStr=boolean  InputSameDT=off
  compare: O_Va : Scope  NumInputPorts=3
  wires:
  Compare To Zero/1 -> compare: O_Va/3  "err"
  Relational Operator/1 -> Compare To Zero/1, AssertEq/1
  cosim/1 -> compare: O_Va/1, Relational Operator/1  "cosim"
  dut/1 -> compare: O_Va/2, Relational Operator/2  "dut ref"

== system gm_HDL_pfc_gold_fi_og_vnl/Compare/Assert_O_Vb ==
  cosim : Inport
  dut : Inport  Port=2
  AssertEq : Assertion  StopWhenAssertionFail=off
  Compare To Zero : simulink/Logic and Bit Operations/Compare To Zero  relop===  OutDataTypeStr=boolean
  Relational Operator : RelationalOperator  Operator===  OutDataTypeStr=boolean  InputSameDT=off
  compare: O_Vb : Scope  NumInputPorts=3
  wires:
  Compare To Zero/1 -> compare: O_Vb/3  "err"
  Relational Operator/1 -> Compare To Zero/1, AssertEq/1
  cosim/1 -> compare: O_Vb/1, Relational Operator/1  "cosim"
  dut/1 -> compare: O_Vb/2, Relational Operator/2  "dut ref"

== system gm_HDL_pfc_gold_fi_og_vnl/Compare/Assert_O_Vc ==
  cosim : Inport
  dut : Inport  Port=2
  AssertEq : Assertion  StopWhenAssertionFail=off
  Compare To Zero : simulink/Logic and Bit Operations/Compare To Zero  relop===  OutDataTypeStr=boolean
  Relational Operator : RelationalOperator  Operator===  OutDataTypeStr=boolean  InputSameDT=off
  compare: O_Vc : Scope  NumInputPorts=3
  wires:
  Compare To Zero/1 -> compare: O_Vc/3  "err"
  Relational Operator/1 -> Compare To Zero/1, AssertEq/1
  cosim/1 -> compare: O_Vc/1, Relational Operator/1  "cosim"
  dut/1 -> compare: O_Vc/2, Relational Operator/2  "dut ref"

== system gm_HDL_pfc_gold_fi_og_vnl/Compare/Assert_O_Vout ==
  cosim : Inport
  dut : Inport  Port=2
  AssertEq : Assertion  StopWhenAssertionFail=off
  Compare To Zero : simulink/Logic and Bit Operations/Compare To Zero  relop===  OutDataTypeStr=boolean
  Relational Operator : RelationalOperator  Operator===  OutDataTypeStr=boolean  InputSameDT=off
  compare: O_Vout : Scope  NumInputPorts=3
  wires:
  Compare To Zero/1 -> compare: O_Vout/3  "err"
  Relational Operator/1 -> Compare To Zero/1, AssertEq/1
  cosim/1 -> compare: O_Vout/1, Relational Operator/1  "cosim"
  dut/1 -> compare: O_Vout/2, Relational Operator/2  "dut ref"

== system gm_HDL_pfc_gold_fi_og_vnl/Compare/CleanupScopes ==

== system gm_HDL_pfc_gold_fi_og_vnl/Compare/Enable ==

== system gm_HDL_pfc_gold_fi_og_vnl/Subsystem1/ctrl_pwm ==
  a : Inport
  b : Inport  Port=2
  O_Va : Inport  Port=3
  O_Vb : Inport  Port=4
  O_Vc : Inport  Port=5
  Enable : EnablePort
  PI_CTRL : Subsystem
  SVPWM : Subsystem
  transforms : Subsystem
  Qs : Outport
  wires:
  transforms/1(id) -> PI_CTRL/1(id)
  transforms/3(angle) -> SVPWM/2(angle)
  PI_CTRL/1(Vd_inductor) -> SVPWM/1(Vd_inductor)
  a/1 -> transforms/1(a)
  O_Vc/1 -> transforms/5(In5)
  transforms/2(iq) -> PI_CTRL/2(iq)
  SVPWM/1(P) -> Qs/1  "Qs"
  PI_CTRL/2(Vq_inductor) -> SVPWM/3(Vq_inductor)
  b/1 -> transforms/2(b)
  O_Va/1 -> transforms/3(In3)
  O_Vb/1 -> transforms/4(In4)

== system gm_HDL_pfc_gold_fi_og_vnl/Subsystem1/real2uint8 ==
  Ia : Inport
  Ib : Inport  Port=2
  Va : Inport  Port=3
  Vb : Inport  Port=4
  Vc : Inport  Port=5
  Add2 : Sum  Inputs=-+  OutDataTypeStr=Inherit: Same as first input
  Add3 : Sum  Inputs=+-
  Constant : Constant  Value=40  SampleTime=-1
  Constant1 : Constant  Value=420  SampleTime=-1
  Demux : Demux  Outputs=3
  Demux1 : Demux  Outputs=2
  Gain2 : Gain  Gain=80/nbits  OutDataTypeStr=Inherit: Same as input
  Gain5 : Gain  Gain=840/nbits  OutDataTypeStr=Inherit: Same as input
  Mux : Mux  Inputs=3
  Mux1 : Mux  Inputs=2
  O_Ia : Outport
  O_Ib : Outport  Port=2
  O_Va : Outport  Port=3
  O_Vb : Outport  Port=4
  O_Vc : Outport  Port=5
  wires:
  Va/1 -> Mux/3
  Vb/1 -> Mux/1
  Ia/1 -> Mux1/2  "rIA"
  Vc/1 -> Mux/2
  Ib/1 -> Mux1/1
  Demux/1 -> O_Vb/1
  Constant1/1 -> Add3/2
  Constant/1 -> Add2/1
  Demux/2 -> O_Vc/1
  Demux/3 -> O_Va/1
  Demux1/1 -> O_Ib/1
  Demux1/2 -> O_Ia/1
  Mux1/1 -> Gain2/1
  Mux/1 -> Gain5/1
  Gain5/1 -> Add3/1
  Gain2/1 -> Add2/2
  Add2/1 -> Demux1/1
  Add3/1 -> Demux/1

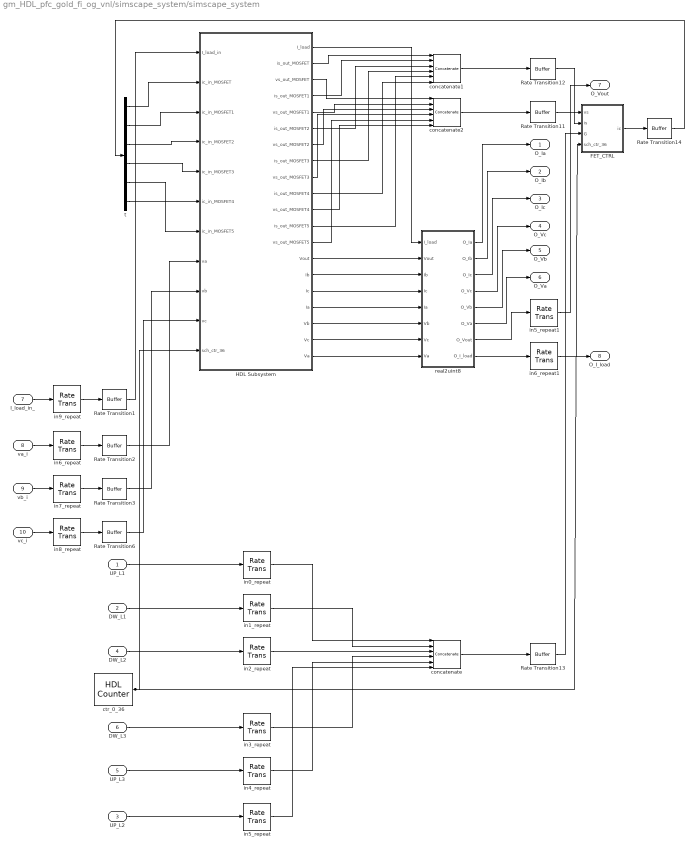
== system gm_HDL_pfc_gold_fi_og_vnl/simscape_system/simscape_system ==
  UP_L1 : Inport  OutDataTypeStr=boolean  SampleTime=5.12820512820513e-07
  DW_L1 : Inport  Port=2  OutDataTypeStr=boolean  SampleTime=5.12820512820513e-07
  UP_L2 : Inport  Port=3  OutDataTypeStr=boolean  SampleTime=5.12820512820513e-07
  DW_L2 : Inport  Port=4  OutDataTypeStr=boolean  SampleTime=5.12820512820513e-07
  UP_L3 : Inport  Port=5  OutDataTypeStr=boolean  SampleTime=5.12820512820513e-07
  DW_L3 : Inport  Port=6  OutDataTypeStr=boolean  SampleTime=5.12820512820513e-07
  I_load_in_ : Inport  Port=7  OutDataTypeStr=fixdt(1, 18, 8)  SampleTime=5.12820512820513e-07
  va_i : Inport  Port=8  OutDataTypeStr=fixdt(1, 18, 8)  SampleTime=5.12820512820513e-07
  vb_i : Inport  Port=9  OutDataTypeStr=fixdt(1, 18, 8)  SampleTime=5.12820512820513e-07
  vc_i : Inport  Port=10  OutDataTypeStr=fixdt(1, 18, 8)  SampleTime=5.12820512820513e-07
  FET_CTRL : Subsystem
  HDL Subsystem : Subsystem
  Rate Transition{1..3,6,11..14} (8 alike) : hdlmdlgenlib/Buffer
  concatenate : Concatenate  NumInputs=6
  concatenate1 : Concatenate  NumInputs=6
  concatenate2 : Concatenate  NumInputs=6
  ctr_0_36 : hdlsllib/Sources/HDL Counter  CountType=Count limited  CountInit=double(0)  CountStep=double(1)  CountMax=double(36)  CountFromType=Initial value  CountFrom=double(0)  CountResetPort=off  CountLoadPort=off  CountEnbPort=off  CountDirPort=off  CountHitOutputPort=off  CountDataType=Unsigned  CountWordLen=6  CountFracLen=0  CountSampTime=1.38600138600139e-08
  in0_repeat : RateTransition  Integrity=off  Deterministic=off  OutPortSampleTimeOpt=Multiple of input port sample time  OutPortSampleTimeMultiple=1/37
  in1_repeat : RateTransition  Integrity=off  Deterministic=off  OutPortSampleTimeOpt=Multiple of input port sample time  OutPortSampleTimeMultiple=1/37
  in2_repeat : RateTransition  Integrity=off  Deterministic=off  OutPortSampleTimeOpt=Multiple of input port sample time  OutPortSampleTimeMultiple=1/37
  in3_repeat : RateTransition  Integrity=off  Deterministic=off  OutPortSampleTimeOpt=Multiple of input port sample time  OutPortSampleTimeMultiple=1/37
  in4_repeat : RateTransition  Integrity=off  Deterministic=off  OutPortSampleTimeOpt=Multiple of input port sample time  OutPortSampleTimeMultiple=1/37
  in5_repeat : RateTransition  Integrity=off  Deterministic=off  OutPortSampleTimeOpt=Multiple of input port sample time  OutPortSampleTimeMultiple=1/37
  in5_repeat1 : RateTransition  Integrity=off  Deterministic=off  OutPortSampleTimeOpt=Multiple of input port sample time  OutPortSampleTimeMultiple=1/37
  in6_repeat : RateTransition  Integrity=off  Deterministic=off  OutPortSampleTimeOpt=Multiple of input port sample time  OutPortSampleTimeMultiple=1/37
  in6_repeat1 : RateTransition  Integrity=off  Deterministic=off  OutPortSampleTimeOpt=Multiple of input port sample time  OutPortSampleTimeMultiple=1/37
  in7_repeat : RateTransition  Integrity=off  Deterministic=off  OutPortSampleTimeOpt=Multiple of input port sample time  OutPortSampleTimeMultiple=1/37
  in8_repeat : RateTransition  Integrity=off  Deterministic=off  OutPortSampleTimeOpt=Multiple of input port sample time  OutPortSampleTimeMultiple=1/37
  in9_repeat : RateTransition  Integrity=off  Deterministic=off  OutPortSampleTimeOpt=Multiple of input port sample time  OutPortSampleTimeMultiple=1/37
  real2uint8 : Subsystem
  t : Demux  Outputs=6
  O_Ia : Outport  OutDataTypeStr=fixdt(0, 12, -1)  SampleTime=1.38600138600139e-08
  O_Ib : Outport  Port=2  OutDataTypeStr=fixdt(0, 12, -1)  SampleTime=1.38600138600139e-08
  O_Ic : Outport  Port=3  OutDataTypeStr=fixdt(0, 12, -1)  SampleTime=1.38600138600139e-08
  O_Vc : Outport  Port=4  OutDataTypeStr=fixdt(0, 12, -1)  SampleTime=1.38600138600139e-08
  O_Vb : Outport  Port=5  OutDataTypeStr=fixdt(0, 12, -1)  SampleTime=1.38600138600139e-08
  O_Va : Outport  Port=6  OutDataTypeStr=fixdt(0, 12, -1)  SampleTime=1.38600138600139e-08
  O_Vout : Outport  Port=7  OutDataTypeStr=fixdt(0, 12, -1)  SampleTime=1.38600138600139e-08
  O_I_load : Outport  Port=8  OutDataTypeStr=fixdt(0, 12, -1)  SampleTime=1.38600138600139e-08
  wires:
  Rate Transition14/1 -> t/1
  FET_CTRL/1(ic) -> Rate Transition14/1
  Rate Transition13/1 -> FET_CTRL/3(G)
  in6_repeat1/1 -> O_I_load/1
  in5_repeat1/1 -> O_Vout/1
  concatenate/1 -> Rate Transition13/1
  real2uint8/7(O_Vout) -> in5_repeat1/1
  real2uint8/2(O_Ib) -> O_Ib/1
  real2uint8/1(O_Ia) -> O_Ia/1
  in4_repeat/1 -> concatenate/5
  in3_repeat/1 -> concatenate/4
  in2_repeat/1 -> concatenate/3
  HDL Subsystem/20(Va) -> real2uint8/8(Va)
  HDL Subsystem/18(Vb) -> real2uint8/6(Vb)
  HDL Subsystem/19(Vc) -> real2uint8/7(Vc)
  HDL Subsystem/17(Ia) -> real2uint8/5(Ia)
  HDL Subsystem/16(Ic) -> real2uint8/4(Ic)
  HDL Subsystem/14(Vout) -> real2uint8/2(Vout)
  real2uint8/5(O_Vb) -> O_Vb/1
  HDL Subsystem/13(vs_out_MOSFET5) -> concatenate2/5
  HDL Subsystem/12(is_out_MOSFET5) -> concatenate1/5
  HDL Subsystem/11(vs_out_MOSFET4) -> concatenate2/6
  HDL Subsystem/10(is_out_MOSFET4) -> concatenate1/6
  real2uint8/8(O_I_load) -> in6_repeat1/1
  HDL Subsystem/8(is_out_MOSFET3) -> concatenate1/4
  HDL Subsystem/7(vs_out_MOSFET2) -> concatenate2/3
  HDL Subsystem/9(vs_out_MOSFET3) -> concatenate2/4
  concatenate1/1 -> Rate Transition12/1
  HDL Subsystem/5(vs_out_MOSFET1) -> concatenate2/2
  HDL Subsystem/3(vs_out_MOSFET) -> concatenate2/1
  HDL Subsystem/2(is_out_MOSFET) -> concatenate1/1
  HDL Subsystem/1(I_load) -> real2uint8/1(I_load)
  real2uint8/6(O_Va) -> O_Va/1
  UP_L2/1 -> in5_repeat/1
  UP_L3/1 -> in4_repeat/1
  DW_L3/1 -> in3_repeat/1
  HDL Subsystem/6(is_out_MOSFET2) -> concatenate1/3
  ctr_0_36/1 -> HDL Subsystem/11(sch_ctr_36), FET_CTRL/4(sch_ctr_36)
  DW_L2/1 -> in2_repeat/1
  UP_L1/1 -> in0_repeat/1
  Rate Transition6/1 -> HDL Subsystem/10(vc)
  Rate Transition1/1 -> HDL Subsystem/1(I_load_in)
  t/6 -> HDL Subsystem/6(ic_in_MOSFET4)
  t/5 -> HDL Subsystem/7(ic_in_MOSFET5)
  in1_repeat/1 -> concatenate/2
  t/4 -> HDL Subsystem/5(ic_in_MOSFET3)
  real2uint8/4(O_Vc) -> O_Vc/1
  t/3 -> HDL Subsystem/4(ic_in_MOSFET2)
  t/2 -> HDL Subsystem/3(ic_in_MOSFET1)
  Rate Transition2/1 -> HDL Subsystem/8(va)
  t/1 -> HDL Subsystem/2(ic_in_MOSFET)
  concatenate2/1 -> Rate Transition11/1
  in7_repeat/1 -> Rate Transition3/1
  in6_repeat/1 -> Rate Transition2/1
  Rate Transition11/1 -> FET_CTRL/1(vs)
  in9_repeat/1 -> Rate Transition1/1
  Rate Transition3/1 -> HDL Subsystem/9(vb)
  real2uint8/3(O_Ic) -> O_Ic/1
  HDL Subsystem/4(is_out_MOSFET1) -> concatenate1/2
  I_load_in_/1 -> in9_repeat/1
  HDL Subsystem/15(Ib) -> real2uint8/3(Ib)
  Rate Transition12/1 -> FET_CTRL/2(is)
  va_i/1 -> in6_repeat/1
  in0_repeat/1 -> concatenate/1
  in5_repeat/1 -> concatenate/6
  vb_i/1 -> in7_repeat/1
  in8_repeat/1 -> Rate Transition6/1
  vc_i/1 -> in8_repeat/1
  DW_L1/1 -> in1_repeat/1

== system gm_HDL_pfc_gold_fi_og_vnl/simscape_system_vnl/FET_CTRL ==
  vs : Inport  OutDataTypeStr=fixdt(1,18,6)  SampleTime=t_ss
  is : Inport  Port=2  OutDataTypeStr=fixdt(1,18,6)  SampleTime=t_ss
  G : Inport  Port=3  SampleTime=t_ss
  Constant : Constant  Value=-.7  OutDataTypeStr=fixdt(1,18,17)  SampleTime=t_ss
  Delay : Delay  Commented=through  DelayLength=1  InputProcessing=Columns as channels (frame based)  SampleTime=t_ss
  Delay1 : Delay  Commented=through  DelayLength=1  InputProcessing=Columns as channels (frame based)  SampleTime=t_ss
  Delay2 : Delay  Commented=through  DelayLength=1  InputProcessing=Columns as channels (frame based)  SampleTime=t_ss
  Delay3 : Delay  Commented=through  DelayLength=1  InitialCondition=-.7  InputProcessing=Columns as channels (frame based)  SampleTime=t_ss
  Discrete-Time Integrator : DiscreteIntegrator  IntegratorMethod=Accumulation: Forward Euler  gainval=1/s  SampleTime=t_ss  OutDataTypeStr=fixdt(1,18,8)  SaturateOnIntegerOverflow=on  LimitOutput=on  UpperSaturationLimit=100  LowerSaturationLimit=-100  ICPrevOutput=DiscIntNeverNeededParam  ICPrevScaledInput=DiscIntNeverNeededParam
  Equal : RelationalOperator  OutDataTypeStr=boolean  RndMeth=Simplest  InputSameDT=off
  Gain1 : Gain  Gain=-1  OutDataTypeStr=fixdt(1,18,12)
  Gain3 : Gain  Gain=Gs  OutDataTypeStr=fixdt(1,18,12)
  Multiply-Add : hdlsllib/HDL Operations/Multiply-Add  Function=c+(a.*b)  datatype=fixdt(1,18,12)  DoSatur=on  FMA=off
  OR : Logic  Operator=OR  IconShape=distinctive  AllPortsSameDT=off  OutDataTypeStr=boolean
  Rate Transition{1..5,11} (6 alike) : RateTransition  Commented=through  OutPortSampleTime=t_ss
  Subtract : Sum  Inputs=+-  OutDataTypeStr=fixdt(1,18,12)
  Subtract1 : Sum  Inputs=+-  OutDataTypeStr=fixdt(1,18,11)
  ic : Outport  SampleTime=t_ss
  wires:
  Rate Transition5/1 -> Subtract1/2, Multiply-Add/3
  Rate Transition4/1 -> Multiply-Add/2
  Rate Transition3/1 -> Subtract1/1
  Delay3/1 -> Equal/1
  Rate Transition2/1 -> Equal/2, Gain3/1
  Rate Transition1/1 -> OR/1
  Rate Transition11/1 -> Gain1/1
  Delay2/1 -> Rate Transition2/1
  Delay1/1 -> Rate Transition1/1
  Delay/1 -> Rate Transition11/1
  vs/1 -> Delay2/1
  G/1 -> Delay1/1
  is/1 -> Delay/1
  Multiply-Add/1 -> Subtract/1
  Gain1/1 -> Rate Transition3/1  "on"
  Discrete-Time Integrator/1 -> Subtract/2, ic/1  "ic"
  Subtract/1 -> Discrete-Time Integrator/1
  Equal/1 -> OR/2
  Constant/1 -> Delay3/1
  Gain3/1 -> Rate Transition5/1
  Subtract1/1 -> Multiply-Add/1
  OR/1 -> Rate Transition4/1

== system gm_HDL_pfc_gold_fi_og_vnl/simscape_system_vnl/HDL Subsystem ==
  I_load_in : Inport  OutDataTypeStr=fixdt(1,18,8)
  ic_in_MOSFET : Inport  Port=2  OutDataTypeStr=fixdt(1,18,8)
  ic_in_MOSFET1 : Inport  Port=3  OutDataTypeStr=fixdt(1,18,8)
  ic_in_MOSFET2 : Inport  Port=4  OutDataTypeStr=fixdt(1,18,8)
  ic_in_MOSFET3 : Inport  Port=5  OutDataTypeStr=fixdt(1,18,8)
  ic_in_MOSFET4 : Inport  Port=6  OutDataTypeStr=fixdt(1,18,8)
  ic_in_MOSFET5 : Inport  Port=7  OutDataTypeStr=fixdt(1,18,8)
  va : Inport  Port=8  OutDataTypeStr=fixdt(1,18,8)
  vb : Inport  Port=9  OutDataTypeStr=fixdt(1,18,8)
  vc : Inport  Port=10  OutDataTypeStr=fixdt(1,18,8)
  Data Type Conversion : DataTypeConversion  SaturateOnIntegerOverflow=off  RndMeth=Floor
  Data Type Conversion1 : DataTypeConversion  OutDataTypeStr=fixdt(1,18,6)  SaturateOnIntegerOverflow=off  RndMeth=Floor
  Fixed-Point State-Space : simulink/Additional Math & Discrete/Additional Discrete/Fixed-Point State-Space  A=fi(stateSpaceParameters_1.Ad,1,25,24)  B=fi(stateSpaceParameters_1.Bd,1,25,31)  C=fi(stateSpaceParameters_1.Cd,1,25,20)  D=fi(stateSpaceParameters_1.Dd,1,25,19)  InitialCondition=fi(stateSpaceParameters_1.X0,1,25,14)  InternalDataType=fixdt(1,25,13)  StateEqScaling=2^0  OutputEqScaling=2^0  DoSatur=off
  HDL Algorithm : Subsystem  Commented=on
  Input Concat : Concatenate  NumInputs=10
  Output Demux : Demux  Outputs=20
  I_load : Outport
  is_out_MOSFET : Outport  Port=2
  vs_out_MOSFET : Outport  Port=3
  is_out_MOSFET1 : Outport  Port=4
  vs_out_MOSFET1 : Outport  Port=5
  is_out_MOSFET2 : Outport  Port=6
  vs_out_MOSFET2 : Outport  Port=7
  is_out_MOSFET3 : Outport  Port=8
  vs_out_MOSFET3 : Outport  Port=9
  is_out_MOSFET4 : Outport  Port=10
  vs_out_MOSFET4 : Outport  Port=11
  is_out_MOSFET5 : Outport  Port=12
  vs_out_MOSFET5 : Outport  Port=13
  Vout : Outport  Port=14
  Ib : Outport  Port=15
  Ic : Outport  Port=16
  Ia : Outport  Port=17
  Vb : Outport  Port=18
  Vc : Outport  Port=19
  Va : Outport  Port=20
  wires:
  Fixed-Point State-Space/1 -> Data Type Conversion1/1
  Data Type Conversion/1 -> HDL Algorithm/1(In1), Fixed-Point State-Space/1
  Data Type Conversion1/1 -> Output Demux/1
  ic_in_MOSFET4/1 -> Input Concat/6
  va/1 -> Input Concat/8
  ic_in_MOSFET5/1 -> Input Concat/7
  ic_in_MOSFET2/1 -> Input Concat/4
  ic_in_MOSFET3/1 -> Input Concat/5
  I_load_in/1 -> Input Concat/1  "i_load_in"
  ic_in_MOSFET1/1 -> Input Concat/3
  vb/1 -> Input Concat/9
  Output Demux/20 -> Va/1  "Va"
  Output Demux/18 -> Vb/1  "Vb"
  Output Demux/19 -> Vc/1  "Vc"
  Output Demux/16 -> Ic/1  "Ic"
  Output Demux/14 -> Vout/1  "Vout"
  Output Demux/11 -> vs_out_MOSFET4/1  "vs_out_MOSFET4"
  Output Demux/9 -> vs_out_MOSFET3/1  "vs_out_MOSFET3"
  Output Demux/10 -> is_out_MOSFET4/1  "is_out_MOSFET4"
  Output Demux/12 -> is_out_MOSFET5/1  "is_out_MOSFET5"
  Output Demux/5 -> vs_out_MOSFET1/1  "vs_out_MOSFET1"
  Output Demux/13 -> vs_out_MOSFET5/1  "vs_out_MOSFET5"
  Output Demux/15 -> Ib/1  "Ib"
  Output Demux/8 -> is_out_MOSFET3/1  "is_out_MOSFET3"
  Output Demux/6 -> is_out_MOSFET2/1  "is_out_MOSFET2"
  vc/1 -> Input Concat/10
  Output Demux/1 -> I_load/1  "I_load"
  Output Demux/17 -> Ia/1  "Ia"
  Input Concat/1 -> Data Type Conversion/1
  ic_in_MOSFET/1 -> Input Concat/2
  Output Demux/4 -> is_out_MOSFET1/1  "is_out_MOSFET1"
  Output Demux/3 -> vs_out_MOSFET/1  "vs_out_MOSFET"
  Output Demux/2 -> is_out_MOSFET/1  "is_out_MOSFET"
  Output Demux/7 -> vs_out_MOSFET2/1  "vs_out_MOSFET2"

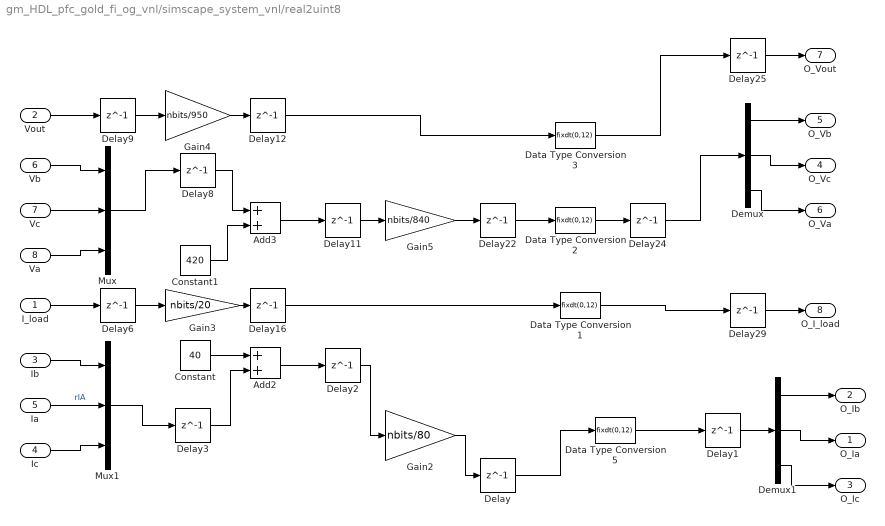
== system gm_HDL_pfc_gold_fi_og_vnl/simscape_system_vnl/real2uint8 ==
  I_load : Inport
  Vout : Inport  Port=2
  Ib : Inport  Port=3
  Ic : Inport  Port=4
  Ia : Inport  Port=5
  Vb : Inport  Port=6
  Vc : Inport  Port=7
  Va : Inport  Port=8
  Add2 : Sum
  Add3 : Sum
  Constant : Constant  Value=40  OutDataTypeStr=fixdt(1,18,6)  SampleTime=-1
  Constant1 : Constant  Value=420  OutDataTypeStr=fixdt(1,18,6)  SampleTime=-1
  Data Type Conversion1 : DataTypeConversion  OutMax=2^12  OutDataTypeStr=fixdt(0,12)  SaturateOnIntegerOverflow=off  RndMeth=Floor  LockScale=on
  Data Type Conversion2 : DataTypeConversion  OutMax=2^12  OutDataTypeStr=fixdt(0,12)  SaturateOnIntegerOverflow=off  RndMeth=Floor  LockScale=on
  Data Type Conversion3 : DataTypeConversion  OutMax=2^12  OutDataTypeStr=fixdt(0,12)  SaturateOnIntegerOverflow=off  RndMeth=Floor  LockScale=on
  Data Type Conversion5 : DataTypeConversion  OutMin=[0]  OutMax=2^12  OutDataTypeStr=fixdt(0,12)  SaturateOnIntegerOverflow=off  RndMeth=Floor  LockScale=on
  Delay{,1..3,6,8..9,11..12,16,22,24..25,29} (14 alike) : Delay  DelayLength=1
  Demux : Demux  Outputs=3
  Demux1 : Demux  Outputs=3
  Gain2 : Gain  Gain=nbits/80
  Gain3 : Gain  Gain=nbits/20
  Gain4 : Gain  Gain=nbits/950
  Gain5 : Gain  Gain=nbits/840
  Mux : Mux  Inputs=3
  Mux1 : Mux  Inputs=3
  O_Ia : Outport
  O_Ib : Outport  Port=2
  O_Ic : Outport  Port=3
  O_Vc : Outport  Port=4
  O_Vb : Outport  Port=5
  O_Va : Outport  Port=6
  O_Vout : Outport  Port=7
  O_I_load : Outport  Port=8
  wires:
  Demux1/2 -> O_Ia/1
  Demux1/1 -> O_Ib/1
  Demux1/3 -> O_Ic/1
  Demux/3 -> O_Va/1
  Demux/2 -> O_Vc/1
  Delay1/1 -> Demux1/1
  Data Type Conversion5/1 -> Delay1/1
  Data Type Conversion2/1 -> Delay24/1
  Delay/1 -> Data Type Conversion5/1
  Delay24/1 -> Demux/1
  Delay22/1 -> Data Type Conversion2/1
  Gain2/1 -> Delay/1
  Delay25/1 -> O_Vout/1
  Data Type Conversion1/1 -> Delay29/1
  Delay16/1 -> Data Type Conversion1/1
  Add3/1 -> Delay11/1
  Delay12/1 -> Data Type Conversion3/1
  Delay3/1 -> Add2/2
  Constant/1 -> Add2/1
  Gain3/1 -> Delay16/1
  Constant1/1 -> Add3/2
  Delay8/1 -> Add3/1
  Delay2/1 -> Gain2/1
  Gain4/1 -> Delay12/1
  Mux1/1 -> Delay3/1
  Delay6/1 -> Gain3/1
  Mux/1 -> Delay8/1
  Delay9/1 -> Gain4/1
  Delay29/1 -> O_I_load/1
  Demux/1 -> O_Vb/1
  I_load/1 -> Delay6/1
  Delay11/1 -> Gain5/1
  Ib/1 -> Mux1/1
  Vc/1 -> Mux/2
  Gain5/1 -> Delay22/1
  Ia/1 -> Mux1/2  "rIA"
  Vb/1 -> Mux/1
  Vout/1 -> Delay9/1
  Data Type Conversion3/1 -> Delay25/1
  Ic/1 -> Mux1/3
  Va/1 -> Mux/3
  Add2/1 -> Delay2/1
